simulink model "seglinear"  (R2020a)
settings: Solver=VariableStepAuto  StartTime=0.0  StopTime=t_stop  RelTol=1e-3
values from neighbouring files (symbols this model uses):
  B = zeros(n,1)    [GetLinModFtxu.m]
  K_lqr = lqr(A,B,Q,R)    [segway_m.m]
  X0 = [0; 0; 2*pi/180; 0]    [segway_m.m]
undefined symbols (not defined in the file or in its folder): A
settings Model: Creator=super  LastModifiedBy=super
settings DataIOCC: SaveFormat=Array  SaveOutput=off  SignalLogging=off  DSMLogging=off  SaveTime=off  ReturnWorkspaceOutputs=off

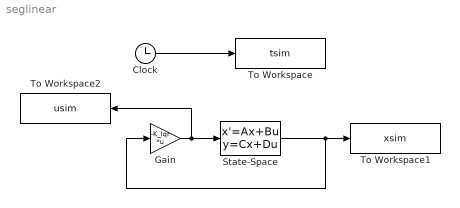
== system seglinear ==
  Clock : Clock
  Gain : Gain  Gain=-K_lqr  Multiplication=Matrix(K*u)
  State-Space : StateSpace  A=A  B=B  C=eye(4,4)  D=zeros(4,1)  InitialCondition=X0
  To Workspace : ToWorkspace  VariableName=tsim  SampleTime=-1
      settings: Save2DSignal=2-D array (concatenate along first dimension)
  To Workspace1 : ToWorkspace  VariableName=xsim  SampleTime=-1
      settings: Save2DSignal=2-D array (concatenate along first dimension)
  To Workspace2 : ToWorkspace  VariableName=usim  SampleTime=-1
      settings: Save2DSignal=2-D array (concatenate along first dimension)
  wires:
  Clock/1 -> To Workspace/1
  Gain/1 -> To Workspace2/1, State-Space/1
  State-Space/1 -> Gain/1, To Workspace1/1
